simulink model "power_BLDC_EGR_Test"  (R2013b)
settings: Solver=FixedStepDiscrete  StartTime=0.0  StopTime=2  FixedStep=Ts  RelTol=1e-3
values from neighbouring files (symbols this model uses):
  C_BLDCM_POLE_NUM = 4    [EGR_Model_Init.m]
  C_BLDCM_ROTOR_RAD_INIT = Simulink.Parameter    [EGR_Model_Init.m]
  C_EGR_BLDC_STEP = 60    [EGR_Model_Init.m]
  C_EGR_BLDC_VALVE_SCREW_LOAD_PITCH = 4    [EGR_Model_Init.m]
  K_BLDCM_DAMPING_COEFF = Simulink.Parameter    [EGR_Model_Init.m]
  K_BLDCM_FLUX = Simulink.Parameter    [EGR_Model_Init.m]
  K_BLDCM_INDUCTANCE = Simulink.Parameter    [EGR_Model_Init.m]
  K_BLDCM_INERTIA = Simulink.Parameter    [EGR_Model_Init.m]
  K_BLDCM_RESISTANCE = Simulink.Parameter    [EGR_Model_Init.m]
  K_BLDCM_TF = Simulink.Parameter    [EGR_Model_Init.m]
  K_EGR_BLDC_LCD_POS_OFFSET = 0    [EGR_Model_Init.m]
  K_EGR_BLDC_VALVE_HS_RAD_HIGH = 15.9082    [EGR_Model_Init.m]
  K_EGR_BLDC_VALVE_HS_RAD_LOW = -3.27    [EGR_Model_Init.m]
  K_EGR_BLDC_VALVE_POS_RAD_INIT = 0    [EGR_Model_Init.m]
  K_EGR_BLDC_VALVE_POS_RAD_OFFSET = 1.047    [EGR_Model_Init.m]
  K_EGR_BLDC_VALVE_STOPPER_RAD = 0.2617    [EGR_Model_Init.m]
  K_EGR_SPRING_COEFF = Simulink.Parameter    [EGR_Model_Init.m]
  K_EGR_SPRING_TORQUE_COMP = 0    [EGR_Model_Init.m]
  Ts = 1e-4    (= 0.0001)    [EGR_Model_Init.m]
undefined symbols (not defined in the file or in its folder): DiscIntNeverNeededParam
settings Model: FPTRunName=FPA_Reference  TunableVars=EGR_BLDC_STEP,Ksp,egr_bldc_initpos,egr_pos_lower_limit,egr_pos_upper_limit,spring_compensation,spring_initpos,spring_maxpos  TunableVarsStorageClass=Auto,Auto,Auto,Auto,Auto,Auto,Auto,Auto  TunableVarsTypeQualifier=,,,,,,,  Creator=stoup_000  LastModifiedBy=TTI1783
settings DataIOCC: ExternalInput=[time2,input2]  SaveFormat=StructureWithTime  SignalLoggingSaveFormat=ModelDataLogs
settings OptimizationCC: InlineParams=on  UseFloatMulNetSlope=on  UseSpecifiedMinMax=on  InlineInvariantSignals=on  EnhancedBackFolding=on  ZeroExternalMemoryAtStartup=off  ZeroInternalMemoryAtStartup=off  EfficientFloat2IntCast=on  OptimizeModelRefInitCode=on  LifeSpan=1  MaxStackSize=64
settings DebuggingCC: MergeDetectMultiDrivingBlocksExec=error  ParameterPrecisionLossMsg=none
settings HardwareCC: ProdLargestAtomicInteger=Long  ProdLargestAtomicFloat=Double  ProdEndianess=LittleEndian  ProdHWDeviceType=ARM Compatible->ARM Cortex
settings RTWCC: SystemTargetFile=ert.tlc  GenCodeOnly=on  GenerateMakefile=off  TemplateMakefile=ert_default_tmf  Description=Embedded Coder  GenerateReport=on  ProcessScript=ert_make_rtw_hook  Toolchain=GNU Tools for ARM Embedded Processors  IncludeHyperlinkInReport=on  LaunchReport=on  GenerateTraceInfo=on  GenerateTraceReport=on  GenerateTraceReportSl=on  GenerateTraceReportSf=on  GenerateTraceReportEml=on  RTWCompilerOptimization=On
settings CodeAppCC: ForceParamTrailComments=on  IgnoreCustomStorageClasses=off  IgnoreTestpoints=on  OperatorAnnotations=on  SimulinkDataObjDesc=on  SFDataObjDesc=on  MATLABFcnDesc=on  InsertBlockDesc=on  MATLABSourceComments=on  EnableCustomComments=on  ReqsInCode=on
settings ERTTargetCC: CodeReplacementLibrary=ANSI_C  GenerateSampleERTMain=on  IncludeMdlTerminateFcn=off  CombineSignalStateStructs=on  SuppressErrorStatus=on  SupportNonFinite=off  ERTCustomFileTemplate=example_file_process.tlc  ConvertIfToSwitch=on  SuppressUnreachableDefaultCases=on

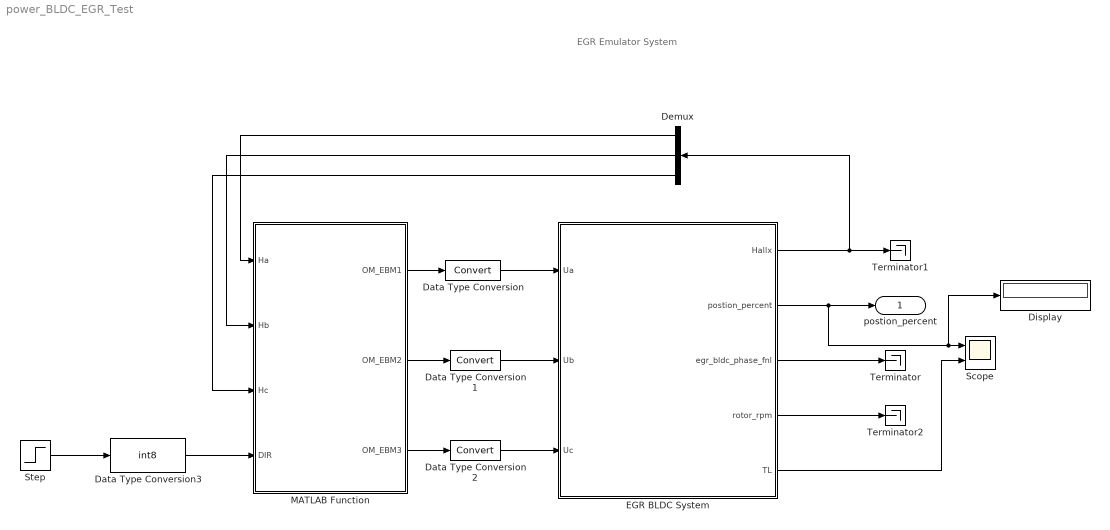
== system power_BLDC_EGR_Test ==
  note: EGR Emulator System
  Data Type Conversion : DataTypeConversion
  Data Type Conversion1 : DataTypeConversion
  Data Type Conversion2 : DataTypeConversion
  Data Type Conversion3 : DataTypeConversion  OutDataTypeStr=int8
  Demux : Demux  Outputs=3
  Display : Display
  EGR BLDC System : Subsystem  MinMaxOverflowLogging=MinMaxAndOverflow
  MATLAB Function : MATLAB Function  TreatAsAtomicUnit=on
  Scope : Scope  NumInputPorts=2
      settings: YMin=-5~-5  YMax=5~5
  Step : Step  Time=.5  Before=1  After=2  SampleTime=0
  Terminator : Terminator
  Terminator1 : Terminator
  Terminator2 : Terminator
  postion_percent : Outport
  wires:
  Data Type Conversion2/1 -> EGR BLDC System/3(Uc)
  Data Type Conversion1/1 -> EGR BLDC System/2(Ub)
  Data Type Conversion/1 -> EGR BLDC System/1(Ua)
  EGR BLDC System/2(postion_percent) -> Display/1, Scope/1, postion_percent/1
  Data Type Conversion3/1 -> MATLAB Function/4(DIR)
  MATLAB Function/1(OM_EBM1) -> Data Type Conversion/1
  MATLAB Function/2(OM_EBM2) -> Data Type Conversion1/1
  MATLAB Function/3(OM_EBM3) -> Data Type Conversion2/1
  EGR BLDC System/3(egr_bldc_phase_fnl) -> Terminator/1
  Demux/1 -> MATLAB Function/1(Ha)
  Demux/2 -> MATLAB Function/2(Hb)
  Demux/3 -> MATLAB Function/3(Hc)
  Step/1 -> Data Type Conversion3/1
  EGR BLDC System/1(Hallx) -> Demux/1, Terminator1/1
  EGR BLDC System/5(TL) -> Scope/2
  EGR BLDC System/4(rotor_rpm) -> Terminator2/1

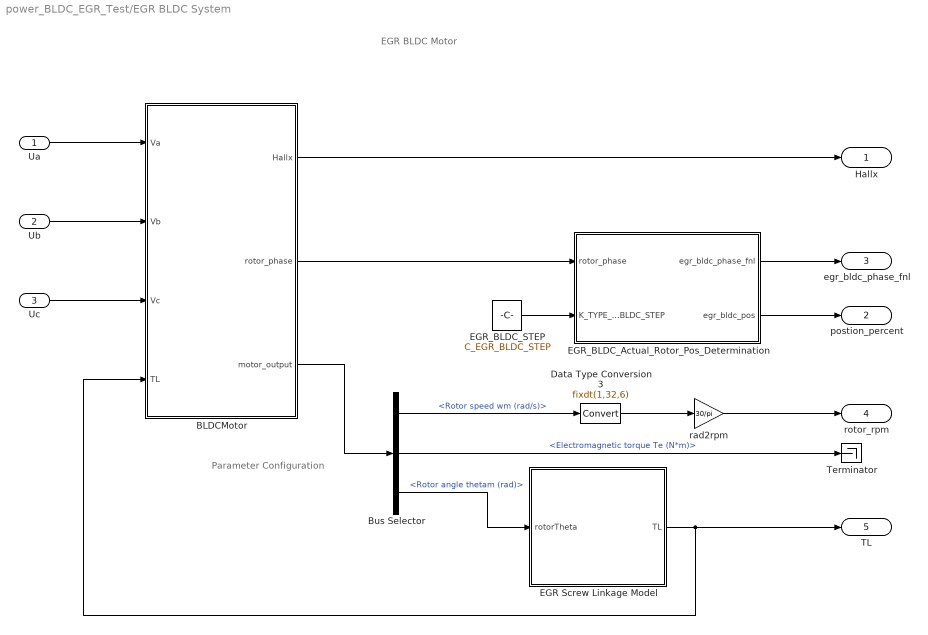
== system power_BLDC_EGR_Test/EGR BLDC System ==
  note: EGR BLDC Motor
  note: Parameter
      | Configuration
  Ua : Inport  OutDataTypeStr=fixdt(1,32,10)
  Ub : Inport  Port=2  OutDataTypeStr=fixdt(1,32,10)
  Uc : Inport  Port=3  OutDataTypeStr=fixdt(1,32,10)
  BLDCMotor : Subsystem
  Bus Selector : BusSelector  OutputSignals=Rotor speed wm (rad/s),Electromagnetic torque Te (N*m),Rotor angle thetam (rad)
  Data Type Conversion3 : DataTypeConversion  OutMin=-2000  OutMax=2000  OutDataTypeStr=fixdt(1,32,6)  RndMeth=Simplest
  EGR Screw Linkage Model : Subsystem  MinMaxOverflowLogging=MinMaxAndOverflow
  EGR_BLDC_Actual_Rotor_Pos_Determination : Subsystem  MinMaxOverflowLogging=MinMaxAndOverflow
  EGR_BLDC_STEP : Constant  Value=C_EGR_BLDC_STEP  OutDataTypeStr=uint8
  Terminator : Terminator
  rad2rpm : Gain  Gain=30/pi  ParamDataTypeStr=fixdt(1,32,10)  OutDataTypeStr=fixdt(1,32,10)  RndMeth=Simplest
  Hallx : Outport
  postion_percent : Outport  Port=2
  egr_bldc_phase_fnl : Outport  Port=3
  rotor_rpm : Outport  Port=4
  TL : Outport  Port=5
  wires:
  EGR Screw Linkage Model/1(TL) -> TL/1, BLDCMotor/4(TL)
  BLDCMotor/1(Hallx) -> Hallx/1
  rad2rpm/1 -> rotor_rpm/1
  Ua/1 -> BLDCMotor/1(Va)
  Ub/1 -> BLDCMotor/2(Vb)
  Uc/1 -> BLDCMotor/3(Vc)
  EGR_BLDC_STEP/1 -> EGR_BLDC_Actual_Rotor_Pos_Determination/2(K_TYPE_EGR_BLDC_STEP)
  EGR_BLDC_Actual_Rotor_Pos_Determination/2(egr_bldc_pos) -> postion_percent/1
  EGR_BLDC_Actual_Rotor_Pos_Determination/1(egr_bldc_phase_fnl) -> egr_bldc_phase_fnl/1
  Data Type Conversion3/1 -> rad2rpm/1
  BLDCMotor/2(rotor_phase) -> EGR_BLDC_Actual_Rotor_Pos_Determination/1(rotor_phase)
  BLDCMotor/3(motor_output) -> Bus Selector/1
  Bus Selector/1 -> Data Type Conversion3/1  "<Rotor speed wm (rad/s)>"
  Bus Selector/2 -> Terminator/1  "<Electromagnetic torque Te (N*m)>"
  Bus Selector/3 -> EGR Screw Linkage Model/1(rotorTheta)  "<Rotor angle thetam (rad)>"

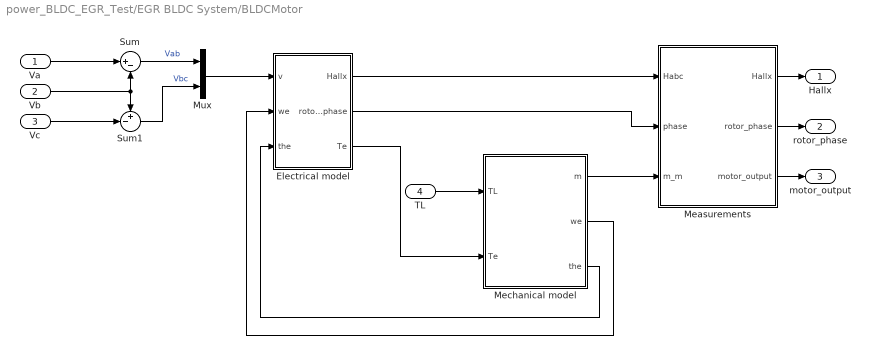
== system power_BLDC_EGR_Test/EGR BLDC System/BLDCMotor ==
  Va : Inport  OutDataTypeStr=fixdt(1,32,10)
  Vb : Inport  Port=2  OutDataTypeStr=fixdt(1,32,10)
  Vc : Inport  Port=3  OutDataTypeStr=fixdt(1,32,10)
  TL : Inport  Port=4  OutDataTypeStr=fixdt(1,32,10)
  Electrical model : Subsystem
  Measurements : Subsystem
  Mechanical model : Subsystem
  Mux : Mux  Inputs=2
  Sum : Sum  Inputs=|+-  OutDataTypeStr=fixdt(1,32,10)
  Sum1 : Sum  Inputs=+-|  OutDataTypeStr=fixdt(1,32,10)
  Hallx : Outport
  rotor_phase : Outport  Port=2
  motor_output : Outport  Port=3
  wires:
  Mechanical model/3(the) -> Electrical model/3(the)
  Mechanical model/1(m) -> Measurements/3(m_m)
  Mux/1 -> Electrical model/1(v)
  TL/1 -> Mechanical model/1(TL)
  Mechanical model/2(we) -> Electrical model/2(we)
  Electrical model/3(Te) -> Mechanical model/2(Te)
  Sum/1 -> Mux/1  "Vab"
  Va/1 -> Sum/1
  Vc/1 -> Sum1/2
  Sum1/1 -> Mux/2  "Vbc"
  Vb/1 -> Sum1/1, Sum/2
  Measurements/1(Hallx) -> Hallx/1
  Electrical model/1(Hallx) -> Measurements/1(Habc)
  Electrical model/2(rotor_phase) -> Measurements/2(phase)
  Measurements/2(rotor_phase) -> rotor_phase/1
  Measurements/3(motor_output) -> motor_output/1

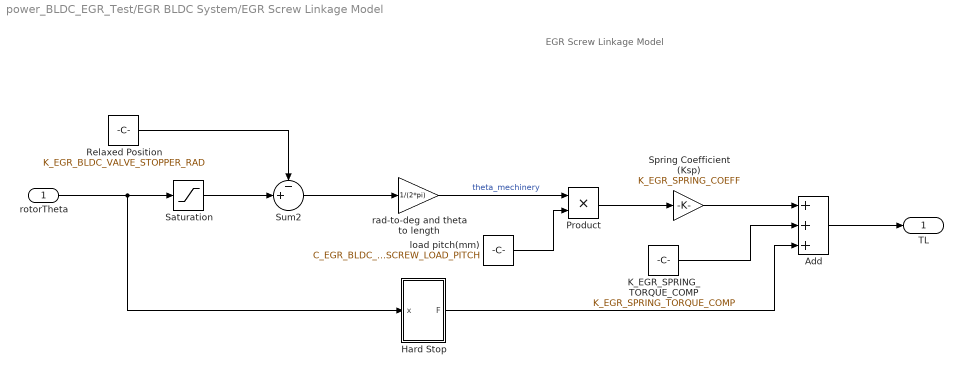
== system power_BLDC_EGR_Test/EGR BLDC System/EGR Screw Linkage Model ==
  note: EGR Screw Linkage Model
  rotorTheta : Inport  OutDataTypeStr=fixdt(1,32,10)
  Add : Sum  Inputs=+++  OutDataTypeStr=fixdt(1,32,10)
  Hard Stop : Subsystem
  K_EGR_SPRING_TORQUE_COMP : Constant  Value=K_EGR_SPRING_TORQUE_COMP  OutDataTypeStr=fixdt(1,32,10)
  Product : Product  OutDataTypeStr=fixdt(1,16,7)
  Relaxed Position : Constant  Value=K_EGR_BLDC_VALVE_STOPPER_RAD  OutDataTypeStr=fixdt(1,32,10)
  Saturation : Saturate  UpperLimit=K_EGR_BLDC_VALVE_HS_RAD_HIGH  LowerLimit=K_EGR_BLDC_VALVE_STOPPER_RAD  OutDataTypeStr=fixdt(1,32,10)
  Spring Coefficient (Ksp) : Gain  Gain=K_EGR_SPRING_COEFF  ParamDataTypeStr=fixdt(1,16,10)  OutDataTypeStr=fixdt(1,16,7)
  Sum2 : Sum  Inputs=-+|  OutDataTypeStr=fixdt(1,32,10)
  load pitch(mm) : Constant  Value=C_EGR_BLDC_VALVE_SCREW_LOAD_PITCH  OutDataTypeStr=fixdt(1,16,7)
  "rad-to-deg and theta to length " : Gain  Gain=1/(2*pi)  ParamDataTypeStr=fixdt(1,32,10)  OutDataTypeStr=fixdt(1,32,10)
  TL : Outport
  wires:
  Spring Coefficient (Ksp)/1 -> Add/1
  rotorTheta/1 -> Hard Stop/1(x), Saturation/1
  Relaxed Position/1 -> Sum2/1
  "rad-to-deg and theta to length "/1 -> Product/1  "theta_mechinery"
  load pitch(mm)/1 -> Product/2
  Sum2/1 -> "rad-to-deg and theta to length "/1
  Product/1 -> Spring Coefficient (Ksp)/1
  K_EGR_SPRING_TORQUE_COMP/1 -> Add/2
  Hard Stop/1(F) -> Add/3
  Add/1 -> TL/1
  Saturation/1 -> Sum2/2

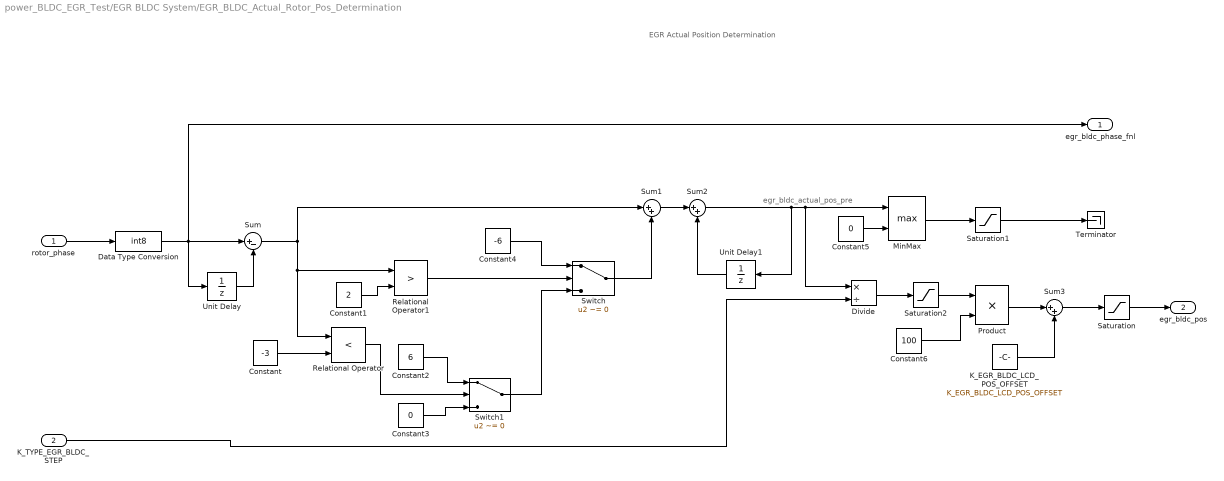
== system power_BLDC_EGR_Test/EGR BLDC System/EGR_BLDC_Actual_Rotor_Pos_Determination ==
  note: EGR Actual Position Determination
  note: egr_bldc_actual_pos_pre
  rotor_phase : Inport  OutDataTypeStr=int8
  K_TYPE_EGR_BLDC_STEP : Inport  Port=2  OutDataTypeStr=uint8
  Constant : Constant  Value=-3  OutDataTypeStr=int8
  Constant1 : Constant  Value=2  OutDataTypeStr=int8
  Constant2 : Constant  Value=6  OutDataTypeStr=int8
  Constant3 : Constant  Value=0  OutDataTypeStr=int8
  Constant4 : Constant  Value=-6  OutDataTypeStr=int8
  Constant5 : Constant  Value=0  OutDataTypeStr=uint8
  Constant6 : Constant  Value=100  OutDataTypeStr=uint8
  Data Type Conversion : DataTypeConversion  OutDataTypeStr=int8
  Divide : Product  Inputs=*/  OutDataTypeStr=fixdt(1,32,12)  RndMeth=Simplest
  K_EGR_BLDC_LCD_POS_OFFSET : Constant  Value=K_EGR_BLDC_LCD_POS_OFFSET  OutDataTypeStr=fixdt(1,16,7)
  MinMax : MinMax  Function=max  Inputs=2  OutDataTypeStr=fixdt(1,16,0)  SaturateOnIntegerOverflow=on
  Product : Product  OutDataTypeStr=fixdt(1,16,7)
  Relational Operator : RelationalOperator  Operator=<  OutDataTypeStr=boolean
  Relational Operator1 : RelationalOperator  Operator=>  OutDataTypeStr=boolean
  Saturation : Saturate  UpperLimit=125  LowerLimit=-25  OutDataTypeStr=fixdt(1,16,7)
  Saturation1 : Saturate  UpperLimit=120  LowerLimit=-60  OutDataTypeStr=int8
  Saturation2 : Saturate  UpperLimit=1.25  LowerLimit=-0.25  OutDataTypeStr=fixdt(1,16,12)
  Sum : Sum  Inputs=|+-  AccumDataTypeStr=int8  OutDataTypeStr=int8
  Sum1 : Sum  Inputs=|++  AccumDataTypeStr=int8  OutDataTypeStr=fixdt(1,8,0)
  Sum2 : Sum  Inputs=|++  AccumDataTypeStr=fixdt(1,16,0)  OutDataTypeStr=fixdt(1,16,0)
  Sum3 : Sum  Inputs=|++  OutDataTypeStr=fixdt(1,16,7)
  Switch : Switch  Criteria=u2 ~= 0  OutDataTypeStr=int8
  Switch1 : Switch  Criteria=u2 ~= 0  OutDataTypeStr=int8
  Terminator : Terminator
  Unit Delay : UnitDelay  SampleTime=-1
  Unit Delay1 : UnitDelay  SampleTime=-1
  egr_bldc_phase_fnl : Outport
  egr_bldc_pos : Outport  Port=2
  wires:
  MinMax/1 -> Saturation1/1
  Switch1/1 -> Switch/3
  Constant4/1 -> Switch/1
  Constant2/1 -> Switch1/1
  Constant/1 -> Relational Operator/2
  Constant3/1 -> Switch1/3
  Constant6/1 -> Product/2
  Relational Operator1/1 -> Switch/2
  Switch/1 -> Sum1/2
  Constant5/1 -> MinMax/2
  Relational Operator/1 -> Switch1/2
  Constant1/1 -> Relational Operator1/2
  Sum1/1 -> Sum2/1
  Unit Delay1/1 -> Sum2/2
  Sum/1 -> Relational Operator/1, Relational Operator1/1, Sum1/1
  Unit Delay/1 -> Sum/2
  Saturation1/1 -> Terminator/1
  K_EGR_BLDC_LCD_POS_OFFSET/1 -> Sum3/2
  Saturation/1 -> egr_bldc_pos/1
  Product/1 -> Sum3/1
  Sum3/1 -> Saturation/1
  Data Type Conversion/1 -> Unit Delay/1, egr_bldc_phase_fnl/1, Sum/1
  Sum2/1 -> Unit Delay1/1, Divide/1, MinMax/1
  rotor_phase/1 -> Data Type Conversion/1
  K_TYPE_EGR_BLDC_STEP/1 -> Divide/2
  Divide/1 -> Saturation2/1
  Saturation2/1 -> Product/1

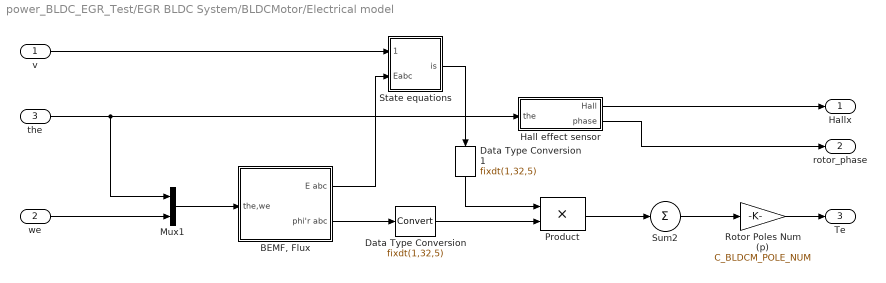
== system power_BLDC_EGR_Test/EGR BLDC System/BLDCMotor/Electrical model ==
  v : Inport
  we : Inport  Port=2
  the : Inport  Port=3
  "BEMF, Flux" : Subsystem
  Data Type Conversion : DataTypeConversion  OutDataTypeStr=fixdt(1,32,5)  RndMeth=Simplest
  Data Type Conversion1 : DataTypeConversion  OutDataTypeStr=fixdt(1,32,5)  RndMeth=Simplest
  Hall effect sensor : Subsystem
  Mux1 : Mux  Inputs=2
  Product : Product  OutDataTypeStr=fixdt(1,32,10)
  Rotor Poles Num (p) : Gain  Gain=C_BLDCM_POLE_NUM  ParamDataTypeStr=int8  OutDataTypeStr=fixdt(1,32,10)
  State equations : Subsystem
  Sum2 : Sum  Inputs=+  OutDataTypeStr=fixdt(1,32,10)  SaturateOnIntegerOverflow=on
  Hallx : Outport  OutDataTypeStr=boolean  InitialOutput=0
  rotor_phase : Outport  Port=2  InitialOutput=0
  Te : Outport  Port=3  OutDataTypeStr=fixdt(1,32,10)  InitialOutput=0
  wires:
  v/1 -> State equations/1(Vab,Vbc)
  Rotor Poles Num (p)/1 -> Te/1
  Sum2/1 -> Rotor Poles Num (p)/1
  "BEMF, Flux"/2(phi'r abc) -> Data Type Conversion/1
  Mux1/1 -> "BEMF, Flux"/1(the,we)
  Product/1 -> Sum2/1
  State equations/1(is) -> Data Type Conversion1/1
  "BEMF, Flux"/1(E abc) -> State equations/2(Eabc)
  we/1 -> Mux1/2
  Data Type Conversion/1 -> Product/2
  Data Type Conversion1/1 -> Product/1
  Hall effect sensor/1(Hall) -> Hallx/1
  Hall effect sensor/2(phase) -> rotor_phase/1
  the/1 -> Hall effect sensor/1(the), Mux1/1

== system power_BLDC_EGR_Test/EGR BLDC System/BLDCMotor/Measurements ==
  Habc : Inport  OutDataTypeStr=boolean
  phase : Inport  Port=2  OutDataTypeStr=int8
  m_m : Inport  Port=3  OutDataTypeStr=fixdt(1,32,10)
  Bus Creator1 : BusCreator  Inputs=3
  Demux1 : Demux  Outputs=[1,1,1]
  Hallx : Outport
  rotor_phase : Outport  Port=2
  motor_output : Outport  Port=3
  wires:
  Demux1/2 -> Bus Creator1/2  "Rotor angle thetam (rad)"
  Demux1/3 -> Bus Creator1/3  "Electromagnetic torque Te (N*m)"
  Demux1/1 -> Bus Creator1/1  "Rotor speed wm (rad/s)"
  m_m/1 -> Demux1/1
  Habc/1 -> Hallx/1
  phase/1 -> rotor_phase/1
  Bus Creator1/1 -> motor_output/1

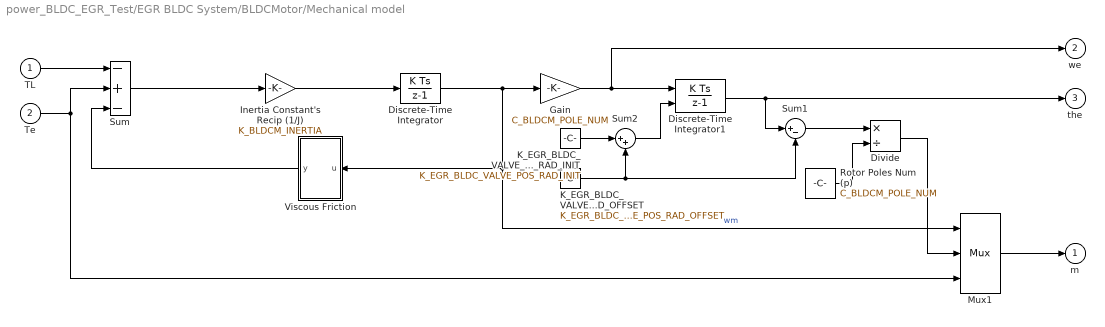
== system power_BLDC_EGR_Test/EGR BLDC System/BLDCMotor/Mechanical model ==
  TL : Inport
  Te : Inport  Port=2  OutDataTypeStr=fixdt(1,32,10)
  Discrete-Time Integrator : DiscreteIntegrator  InitialCondition=C_BLDCM_ROTOR_RAD_INIT  SampleTime=Ts  OutDataTypeStr=fixdt(1,32,10)  ICPrevOutput=DiscIntNeverNeededParam  ICPrevScaledInput=DiscIntNeverNeededParam
  Discrete-Time Integrator1 : DiscreteIntegrator  InitialConditionSource=external  SampleTime=Ts  OutDataTypeStr=fixdt(1,32,10)  ICPrevOutput=DiscIntNeverNeededParam  ICPrevScaledInput=DiscIntNeverNeededParam
  Divide : Product  Inputs=*/  OutDataTypeStr=fixdt(1,32,10)  RndMeth=Simplest
  Gain : Gain  Gain=C_BLDCM_POLE_NUM  ParamMin=0  ParamMax=10  ParamDataTypeStr=int8  OutDataTypeStr=fixdt(1,32,10)
  Inertia Constant's Recip (1/J) : Gain  Gain=K_BLDCM_INERTIA  ParamDataTypeStr=fixdt(1,32,10)  OutDataTypeStr=fixdt(1,32,10)
  K_EGR_BLDC_VALVE_POS_RAD_INIT : Constant  Value=K_EGR_BLDC_VALVE_POS_RAD_INIT  OutDataTypeStr=fixdt(1,32,10)
  K_EGR_BLDC_VALVE_POS_RAD_OFFSET : Constant  Value=K_EGR_BLDC_VALVE_POS_RAD_OFFSET  OutDataTypeStr=fixdt(1,32,10)
  Mux1 : Mux  Inputs=3
  Rotor Poles Num (p) : Constant  Value=C_BLDCM_POLE_NUM  OutDataTypeStr=int8
  Sum : Sum  Inputs=-+-  OutDataTypeStr=fixdt(1,32,10)  SaturateOnIntegerOverflow=on
  Sum1 : Sum  Inputs=|+-  OutDataTypeStr=fixdt(1,32,10)  RndMeth=Simplest
  Sum2 : Sum  Inputs=|++  OutDataTypeStr=fixdt(1,32,10)
  Viscous Friction : Subsystem
  m : Outport  OutDataTypeStr=fixdt(1,32,10)  InitialOutput=0
  we : Outport  Port=2  InitialOutput=0
  the : Outport  Port=3  InitialOutput=0
  wires:
  Te/1 -> Sum/2, Mux1/3
  Gain/1 -> we/1, Discrete-Time Integrator1/1
  Viscous Friction/1(y) -> Sum/3
  TL/1 -> Sum/1
  Discrete-Time Integrator/1 -> Mux1/1, Viscous Friction/1(u), Gain/1  "wm"
  Mux1/1 -> m/1
  Divide/1 -> Mux1/2
  K_EGR_BLDC_VALVE_POS_RAD_OFFSET/1 -> Sum2/2, Sum1/2
  Sum1/1 -> Divide/1
  Sum/1 -> Inertia Constant's Recip (1/J)/1
  Inertia Constant's Recip (1/J)/1 -> Discrete-Time Integrator/1
  Discrete-Time Integrator1/1 -> Sum1/1, the/1
  K_EGR_BLDC_VALVE_POS_RAD_INIT/1 -> Sum2/1
  Sum2/1 -> Discrete-Time Integrator1/2
  Rotor Poles Num (p)/1 -> Divide/2

== system power_BLDC_EGR_Test/EGR BLDC System/EGR Screw Linkage Model/Hard Stop ==
  note: Spring Hard Stop
  x : Inport
  Gain2 : Gain  Gain=800  OutDataTypeStr=fixdt(1,32,10)  ParamDataTypeStr=Inherit: Same as input
  High : Constant  Value=K_EGR_BLDC_VALVE_HS_RAD_HIGH  OutDataTypeStr=fixdt(1,32,10)
  Low : Constant  Value=K_EGR_BLDC_VALVE_HS_RAD_LOW  OutDataTypeStr=fixdt(1,32,10)
  Min1 : MinMax  Inputs=2  OutDataTypeStr=fixdt(1,32,10)  SaturateOnIntegerOverflow=on
  Min3 : MinMax  Function=max  Inputs=2  OutDataTypeStr=fixdt(1,32,10)  SaturateOnIntegerOverflow=on
  Sum5 : Sum  Inputs=-+||+-  OutDataTypeStr=fixdt(1,32,10)  SaturateOnIntegerOverflow=on
  F : Outport
  wires:
  Sum5/1 -> Gain2/1
  x/1 -> Min3/2, Min1/1
  Gain2/1 -> F/1
  Min3/1 -> Sum5/2
  Low/1 -> Sum5/4, Min1/2
  High/1 -> Min3/1, Sum5/1
  Min1/1 -> Sum5/3

== system power_BLDC_EGR_Test/EGR BLDC System/BLDCMotor/Electrical model/BEMF, Flux ==
  the,we : Inport
  Mux4 : Mux  Inputs=3
  Mux7 : Mux  Inputs=3
  Phase a : Subsystem
  Phase b : Subsystem
  Phase c : Subsystem
  E abc : Outport  OutDataTypeStr=fixdt(1,32,10)
  phi'r abc : Outport  Port=2  OutDataTypeStr=fixdt(1,32,10)
  wires:
  Mux7/1 -> phi'r abc/1
  Mux4/1 -> E abc/1
  Phase c/1(phi'r) -> Mux7/3
  Phase b/1(phi'r) -> Mux7/2
  Phase a/1(phi'r) -> Mux7/1
  Phase c/2(E) -> Mux4/3
  Phase b/2(E) -> Mux4/2
  Phase a/2(E) -> Mux4/1
  the,we/1 -> Phase b/1(the,we), Phase a/1(the,we), Phase c/1(the,we)

== system power_BLDC_EGR_Test/EGR BLDC System/BLDCMotor/Electrical model/Hall effect sensor ==
  note: BLDC Motor Hall Encoder
  the : Inport
  S-Function HallDecoder : S-Function  InitFcn=try, set_param(gcb,'FunctionName','HallEncoder'), end  FunctionName=HallEncoder  SFunctionModules=HallEncoder_wrapper  EnableBusSupport=off  mask(S-Function Builder){}
      mask help: Simulink:masks:SFunctionBuilder_MD
      mask init:
      | val = [[.9  0.75 0.75 1 1 .9 .9 1]',[1 1 0.75 0.75 .9 .9 1 .9]'];try , sys = get_param(gcb,'SfunBuilderFcnName');if isempty(sys), sys = get_param(gcb,'FunctionName'); end,catch, sys = get_param(gcb,'FunctionName'); end
      settings: CopyFcn=set_param(gcbh,'LinkStatus','none')  PreSaveFcn=try, set_param(gcb,'FunctionName','HallEncoder'), end  OpenFcn=sfunctionwizard(gcbh)
      mask Display: plot(val(:,1),val(:,2)),disp(sys), port_label('input',1,'theta'), port_label('output',1,'Hallx'), port_label('output',2,'phase')
  rad2deg1 : Gain  Gain=180/pi  OutMin=-360  OutMax=360  OutDataTypeStr=double  RndMeth=Simplest
  rem : Subsystem  TreatAsAtomicUnit=on
  Hall : Outport  OutDataTypeStr=boolean
  phase : Outport  Port=2  OutDataTypeStr=int8
  wires:
  S-Function HallDecoder/1 -> Hall/1
  S-Function HallDecoder/2 -> phase/1
  the/1 -> rem/1(the)
  rem/1(rad) -> rad2deg1/1
  rad2deg1/1 -> S-Function HallDecoder/1

== system power_BLDC_EGR_Test/EGR BLDC System/BLDCMotor/Electrical model/State equations ==
  Vab,Vbc : Inport
  Eabc : Inport  Port=2  OutDataTypeStr=fixdt(1,32,10)
  Mux5 : Mux  Inputs=3
  State Ia : Subsystem
  State Ib : Subsystem
  Sum1 : Sum  Inputs=--  OutDataTypeStr=fixdt(1,32,10)  SaturateOnIntegerOverflow=on
  is : Outport  OutDataTypeStr=fixdt(1,32,10)
  wires:
  Mux5/1 -> is/1
  Eabc/1 -> State Ib/2(Eabc), State Ia/2(Eabc)
  Sum1/1 -> Mux5/3
  State Ia/1(i) -> Sum1/1, Mux5/1
  Vab,Vbc/1 -> State Ib/1(Vab,Vbc), State Ia/1(Vab,Vbc)
  State Ib/1(i) -> Sum1/2, Mux5/2

== system power_BLDC_EGR_Test/EGR BLDC System/BLDCMotor/Mechanical model/Viscous Friction ==
  note: y = sign(x) * (Gain * abs(x) + Offset)
  u : Inport
  Damping Constant (B) : Gain  Gain=K_BLDCM_DAMPING_COEFF  ParamDataTypeStr=fixdt(1,32,10)  OutDataTypeStr=fixdt(1,32,10)
  Shaft static friction torque (Tf) : Gain  Gain=K_BLDCM_TF  ParamDataTypeStr=fixdt(1,32,10)  OutDataTypeStr=fixdt(1,32,10)
  Sign : Signum  DisableCoverage=on
  Sum2 : Sum  Inputs=|++  SaturateOnIntegerOverflow=on  InputSameDT=on  OutDataTypeStr=Inherit: Same as first input
  y : Outport
  wires:
  Damping Constant (B)/1 -> Sum2/2
  Shaft static friction torque (Tf)/1 -> Sum2/1
  Sign/1 -> Shaft static friction torque (Tf)/1
  u/1 -> Damping Constant (B)/1, Sign/1
  Sum2/1 -> y/1

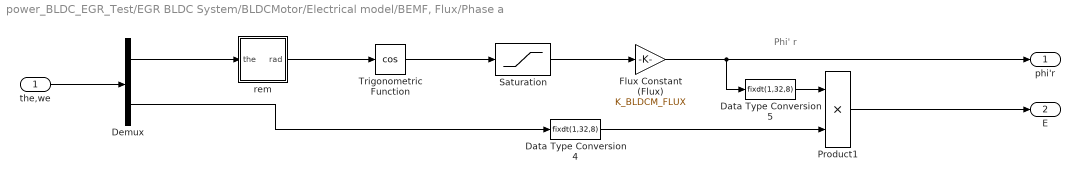
== system power_BLDC_EGR_Test/EGR BLDC System/BLDCMotor/Electrical model/BEMF, Flux/Phase a ==
  note: Phi' r
  the,we : Inport
  Data Type Conversion4 : DataTypeConversion  OutMin=-1000  OutMax=1000  OutDataTypeStr=fixdt(1,32,8)
  Data Type Conversion5 : DataTypeConversion  OutMin=-10  OutMax=10  OutDataTypeStr=fixdt(1,32,8)
  Demux : Demux  Outputs=2
  Flux Constant (Flux) : Gain  Gain=K_BLDCM_FLUX  ParamDataTypeStr=fixdt(1,32,10)  OutDataTypeStr=fixdt(1,32,10)
  Product1 : Product  OutDataTypeStr=fixdt(1,32,10)
  Saturation : Saturate  OutMin=-1  OutMax=1  OutDataTypeStr=fixdt(1,32,10)
  Trigonometric Function : Trigonometry  Operator=cos  ApproximationMethod=CORDIC
  rem : Subsystem  TreatAsAtomicUnit=on
  phi'r : Outport  OutDataTypeStr=fixdt(1,32,10)
  E : Outport  Port=2  OutDataTypeStr=fixdt(1,32,10)
  wires:
  Flux Constant (Flux)/1 -> phi'r/1, Data Type Conversion5/1
  the,we/1 -> Demux/1
  Demux/2 -> Data Type Conversion4/1
  Saturation/1 -> Flux Constant (Flux)/1
  Product1/1 -> E/1
  Data Type Conversion4/1 -> Product1/2
  Data Type Conversion5/1 -> Product1/1
  Demux/1 -> rem/1(the)
  Trigonometric Function/1 -> Saturation/1
  rem/1(rad) -> Trigonometric Function/1

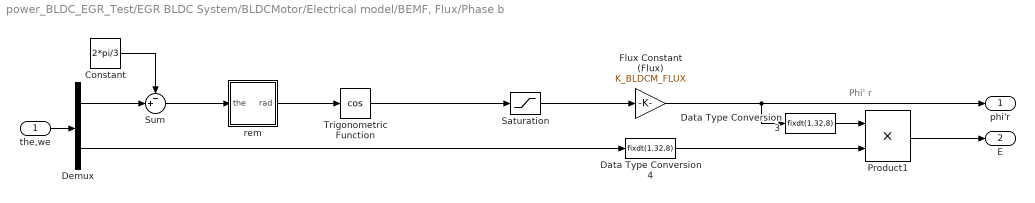
== system power_BLDC_EGR_Test/EGR BLDC System/BLDCMotor/Electrical model/BEMF, Flux/Phase b ==
  note: Phi' r
  the,we : Inport
  Constant : Constant  Value=2*pi/3  OutDataTypeStr=fixdt(1,32,29)
  Data Type Conversion3 : DataTypeConversion  OutMin=-10  OutMax=10  OutDataTypeStr=fixdt(1,32,8)
  Data Type Conversion4 : DataTypeConversion  OutMin=-1000  OutMax=1000  OutDataTypeStr=fixdt(1,32,8)
  Demux : Demux  Outputs=2
  Flux Constant (Flux) : Gain  Gain=K_BLDCM_FLUX  ParamDataTypeStr=fixdt(1,32,10)  OutDataTypeStr=fixdt(1,32,10)
  Product1 : Product  OutDataTypeStr=fixdt(1,32,10)
  Saturation : Saturate  OutMin=-1  OutMax=1  OutDataTypeStr=fixdt(1,32,10)
  Sum : Sum  Inputs=-+|  OutDataTypeStr=fixdt(1,32,10)
  Trigonometric Function : Trigonometry  Operator=cos  ApproximationMethod=CORDIC
  rem : Subsystem  TreatAsAtomicUnit=on
  phi'r : Outport  OutDataTypeStr=fixdt(1,32,10)
  E : Outport  Port=2  OutDataTypeStr=fixdt(1,32,10)
  wires:
  Saturation/1 -> Flux Constant (Flux)/1
  Demux/2 -> Data Type Conversion4/1
  the,we/1 -> Demux/1
  Product1/1 -> E/1
  Flux Constant (Flux)/1 -> phi'r/1, Data Type Conversion3/1
  Constant/1 -> Sum/1
  Demux/1 -> Sum/2
  Data Type Conversion4/1 -> Product1/2
  Data Type Conversion3/1 -> Product1/1
  Trigonometric Function/1 -> Saturation/1
  Sum/1 -> rem/1(the)
  rem/1(rad) -> Trigonometric Function/1

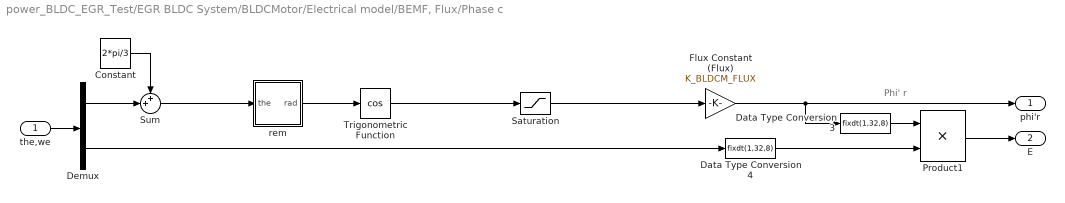
== system power_BLDC_EGR_Test/EGR BLDC System/BLDCMotor/Electrical model/BEMF, Flux/Phase c ==
  note: Phi' r
  the,we : Inport
  Constant : Constant  Value=2*pi/3  OutDataTypeStr=fixdt(1,32,29)
  Data Type Conversion3 : DataTypeConversion  OutMin=-10  OutMax=10  OutDataTypeStr=fixdt(1,32,8)
  Data Type Conversion4 : DataTypeConversion  OutMin=-1000  OutMax=1000  OutDataTypeStr=fixdt(1,32,8)
  Demux : Demux  Outputs=2
  Flux Constant (Flux) : Gain  Gain=K_BLDCM_FLUX  ParamDataTypeStr=fixdt(1,32,10)  OutDataTypeStr=fixdt(1,32,10)
  Product1 : Product  OutDataTypeStr=fixdt(1,32,10)
  Saturation : Saturate  OutMin=-1  OutMax=1  OutDataTypeStr=fixdt(1,32,10)
  Sum : Sum  Inputs=++|  OutDataTypeStr=fixdt(1,32,10)
  Trigonometric Function : Trigonometry  Operator=cos  ApproximationMethod=CORDIC
  rem : Subsystem  TreatAsAtomicUnit=on
  phi'r : Outport  OutDataTypeStr=fixdt(1,32,10)
  E : Outport  Port=2  OutDataTypeStr=fixdt(1,32,10)
  wires:
  Flux Constant (Flux)/1 -> phi'r/1, Data Type Conversion3/1
  Product1/1 -> E/1
  the,we/1 -> Demux/1
  Demux/2 -> Data Type Conversion4/1
  Demux/1 -> Sum/2
  Saturation/1 -> Flux Constant (Flux)/1
  Constant/1 -> Sum/1
  Data Type Conversion4/1 -> Product1/2
  Data Type Conversion3/1 -> Product1/1
  Sum/1 -> rem/1(the)
  Trigonometric Function/1 -> Saturation/1
  rem/1(rad) -> Trigonometric Function/1

== system power_BLDC_EGR_Test/EGR BLDC System/BLDCMotor/Electrical model/Hall effect sensor/rem ==
  the : Inport
  Constant : Constant  Value=2*pi  OutDataTypeStr=double
  Data Type Conversion : DataTypeConversion  OutDataTypeStr=double
  Data Type Conversion1 : DataTypeConversion  OutMin=-2*pi  OutMax=2*pi  OutDataTypeStr=fixdt(1,32,10)  RndMeth=Simplest
  S-Function Builder : S-Function  InitFcn=try, set_param(gcb,'FunctionName','remf'), end  FunctionName=remf  SFunctionModules=remf_wrapper  EnableBusSupport=off  mask(S-Function Builder){}
      mask help: Simulink:masks:SFunctionBuilder_MD
      mask init: same as power_BLDC_EGR_Test/EGR BLDC System/BLDCMotor/Electrical model/Hall effect sensor/S-Function HallDecoder
      settings: CopyFcn=set_param(gcbh,'LinkStatus','none')  PreSaveFcn=try, set_param(gcb,'FunctionName','remf'), end  OpenFcn=sfunctionwizard(gcbh)
      mask Display: plot(val(:,1),val(:,2)),disp(sys), port_label('input',1,'x'), port_label('input',2,'y'), port_label('output',1,'z')
  rad : Outport
  wires:
  Constant/1 -> S-Function Builder/2
  S-Function Builder/1 -> Data Type Conversion1/1
  the/1 -> Data Type Conversion/1
  Data Type Conversion/1 -> S-Function Builder/1
  Data Type Conversion1/1 -> rad/1

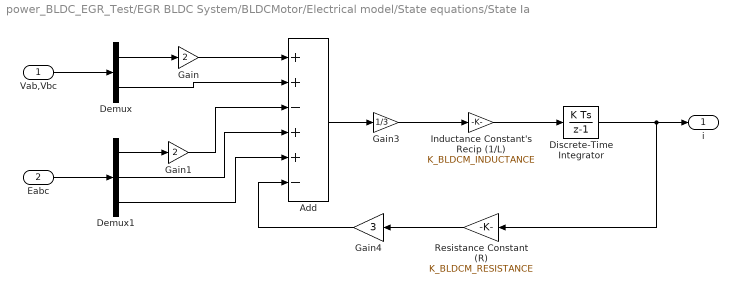
== system power_BLDC_EGR_Test/EGR BLDC System/BLDCMotor/Electrical model/State equations/State Ia ==
  Vab,Vbc : Inport  OutDataTypeStr=fixdt(1,32,10)
  Eabc : Inport  Port=2  OutDataTypeStr=fixdt(1,32,10)
  Add : Sum  Inputs=++-++-  OutDataTypeStr=fixdt(1,32,10)
  Demux : Demux  Outputs=2
  Demux1 : Demux  Outputs=3
  Discrete-Time Integrator : DiscreteIntegrator  SampleTime=Ts  OutDataTypeStr=fixdt(1,32,10)  ICPrevOutput=DiscIntNeverNeededParam  ICPrevScaledInput=DiscIntNeverNeededParam
  Gain : Gain  Gain=2  OutDataTypeStr=fixdt(1,32,10)
  Gain1 : Gain  Gain=2  OutDataTypeStr=fixdt(1,32,10)
  Gain3 : Gain  Gain=1/3  ParamDataTypeStr=fixdt(1,32,10)  OutDataTypeStr=fixdt(1,32,10)
  Gain4 : Gain  Gain=3  OutDataTypeStr=fixdt(1,32,10)  ParamDataTypeStr=Inherit: Same as input
  Inductance Constant's Recip (1/L) : Gain  Gain=K_BLDCM_INDUCTANCE  ParamDataTypeStr=fixdt(1,32,10)  OutDataTypeStr=fixdt(1,32,10)
  Resistance Constant (R) : Gain  Gain=K_BLDCM_RESISTANCE  ParamDataTypeStr=fixdt(1,32,10)  OutDataTypeStr=fixdt(1,32,10)
  i : Outport  OutDataTypeStr=fixdt(1,32,10)
  wires:
  Inductance Constant's Recip (1/L)/1 -> Discrete-Time Integrator/1
  Vab,Vbc/1 -> Demux/1
  Eabc/1 -> Demux1/1
  Demux/1 -> Gain/1
  Gain/1 -> Add/1
  Demux/2 -> Add/2
  Demux1/1 -> Gain1/1
  Gain1/1 -> Add/3
  Demux1/2 -> Add/4
  Demux1/3 -> Add/5
  Resistance Constant (R)/1 -> Gain4/1
  Discrete-Time Integrator/1 -> Resistance Constant (R)/1, i/1
  Add/1 -> Gain3/1
  Gain4/1 -> Add/6
  Gain3/1 -> Inductance Constant's Recip (1/L)/1

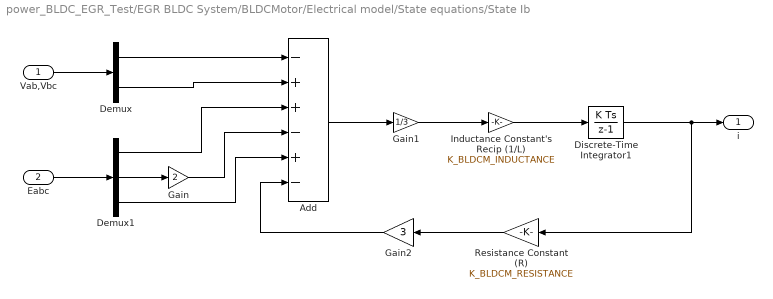
== system power_BLDC_EGR_Test/EGR BLDC System/BLDCMotor/Electrical model/State equations/State Ib ==
  Vab,Vbc : Inport
  Eabc : Inport  Port=2  OutDataTypeStr=fixdt(1,32,10)
  Add : Sum  Inputs=-++-+-  OutDataTypeStr=fixdt(1,32,10)
  Demux : Demux  Outputs=2
  Demux1 : Demux  Outputs=3
  Discrete-Time Integrator1 : DiscreteIntegrator  SampleTime=Ts  OutDataTypeStr=fixdt(1,32,10)  ICPrevOutput=DiscIntNeverNeededParam  ICPrevScaledInput=DiscIntNeverNeededParam
  Gain : Gain  Gain=2  OutDataTypeStr=fixdt(1,32,10)
  Gain1 : Gain  Gain=1/3  ParamDataTypeStr=fixdt(1,32,10)  OutDataTypeStr=fixdt(1,32,10)
  Gain2 : Gain  Gain=3  ParamDataTypeStr=int8  OutDataTypeStr=fixdt(1,32,10)
  Inductance Constant's Recip (1/L) : Gain  Gain=K_BLDCM_INDUCTANCE  ParamDataTypeStr=fixdt(1,32,10)  OutDataTypeStr=fixdt(1,32,10)
  Resistance Constant (R) : Gain  Gain=K_BLDCM_RESISTANCE  ParamDataTypeStr=fixdt(1,32,10)  OutDataTypeStr=fixdt(1,32,10)
  i : Outport  OutDataTypeStr=fixdt(1,32,10)
  wires:
  Vab,Vbc/1 -> Demux/1
  Eabc/1 -> Demux1/1
  Demux/2 -> Add/2
  Demux1/2 -> Gain/1
  Demux1/3 -> Add/5
  Gain2/1 -> Add/6
  Demux/1 -> Add/1
  Demux1/1 -> Add/3
  Gain/1 -> Add/4
  Inductance Constant's Recip (1/L)/1 -> Discrete-Time Integrator1/1
  Add/1 -> Gain1/1
  Discrete-Time Integrator1/1 -> Resistance Constant (R)/1, i/1
  Resistance Constant (R)/1 -> Gain2/1
  Gain1/1 -> Inductance Constant's Recip (1/L)/1

== system power_BLDC_EGR_Test/EGR BLDC System/BLDCMotor/Electrical model/BEMF, Flux/Phase a/rem ==
  the : Inport
  Constant : Constant  Value=2*pi  OutDataTypeStr=double
  Data Type Conversion : DataTypeConversion  OutDataTypeStr=double
  Data Type Conversion1 : DataTypeConversion  OutMin=-2*pi  OutMax=2*pi  OutDataTypeStr=fixdt(1,32,10)  RndMeth=Simplest
  S-Function Builder : S-Function  InitFcn=try, set_param(gcb,'FunctionName','remf'), end  FunctionName=remf  SFunctionModules=remf_wrapper  EnableBusSupport=off  mask(S-Function Builder){}
      mask help: Simulink:masks:SFunctionBuilder_MD
      mask init: same as power_BLDC_EGR_Test/EGR BLDC System/BLDCMotor/Electrical model/Hall effect sensor/S-Function HallDecoder
      settings: CopyFcn=set_param(gcbh,'LinkStatus','none')  PreSaveFcn=try, set_param(gcb,'FunctionName','remf'), end  OpenFcn=sfunctionwizard(gcbh)
      mask Display: plot(val(:,1),val(:,2)),disp(sys), port_label('input',1,'x'), port_label('input',2,'y'), port_label('output',1,'z')
  rad : Outport
  wires:
  Constant/1 -> S-Function Builder/2
  S-Function Builder/1 -> Data Type Conversion1/1
  the/1 -> Data Type Conversion/1
  Data Type Conversion/1 -> S-Function Builder/1
  Data Type Conversion1/1 -> rad/1

== system power_BLDC_EGR_Test/EGR BLDC System/BLDCMotor/Electrical model/BEMF, Flux/Phase b/rem ==
  the : Inport
  Constant : Constant  Value=2*pi  OutDataTypeStr=double
  Data Type Conversion : DataTypeConversion  OutDataTypeStr=double
  Data Type Conversion1 : DataTypeConversion  OutMin=-2*pi  OutMax=2*pi  OutDataTypeStr=fixdt(1,32,10)  RndMeth=Simplest
  S-Function Builder : S-Function  InitFcn=try, set_param(gcb,'FunctionName','remf'), end  FunctionName=remf  SFunctionModules=remf_wrapper  EnableBusSupport=off  mask(S-Function Builder){}
      mask help: Simulink:masks:SFunctionBuilder_MD
      mask init: same as power_BLDC_EGR_Test/EGR BLDC System/BLDCMotor/Electrical model/Hall effect sensor/S-Function HallDecoder
      settings: CopyFcn=set_param(gcbh,'LinkStatus','none')  PreSaveFcn=try, set_param(gcb,'FunctionName','remf'), end  OpenFcn=sfunctionwizard(gcbh)
      mask Display: plot(val(:,1),val(:,2)),disp(sys), port_label('input',1,'x'), port_label('input',2,'y'), port_label('output',1,'z')
  rad : Outport
  wires:
  Constant/1 -> S-Function Builder/2
  S-Function Builder/1 -> Data Type Conversion1/1
  the/1 -> Data Type Conversion/1
  Data Type Conversion/1 -> S-Function Builder/1
  Data Type Conversion1/1 -> rad/1

== system power_BLDC_EGR_Test/EGR BLDC System/BLDCMotor/Electrical model/BEMF, Flux/Phase c/rem ==
  the : Inport
  Constant : Constant  Value=2*pi  OutDataTypeStr=double
  Data Type Conversion : DataTypeConversion  OutDataTypeStr=double
  Data Type Conversion1 : DataTypeConversion  OutMin=-2*pi  OutMax=2*pi  OutDataTypeStr=fixdt(1,32,10)  RndMeth=Simplest
  S-Function Builder : S-Function  InitFcn=try, set_param(gcb,'FunctionName','remf'), end  FunctionName=remf  SFunctionModules=remf_wrapper  EnableBusSupport=off  mask(S-Function Builder){}
      mask help: Simulink:masks:SFunctionBuilder_MD
      mask init: same as power_BLDC_EGR_Test/EGR BLDC System/BLDCMotor/Electrical model/Hall effect sensor/S-Function HallDecoder
      settings: CopyFcn=set_param(gcbh,'LinkStatus','none')  PreSaveFcn=try, set_param(gcb,'FunctionName','remf'), end  OpenFcn=sfunctionwizard(gcbh)
      mask Display: plot(val(:,1),val(:,2)),disp(sys), port_label('input',1,'x'), port_label('input',2,'y'), port_label('output',1,'z')
  rad : Outport
  wires:
  Constant/1 -> S-Function Builder/2
  S-Function Builder/1 -> Data Type Conversion1/1
  the/1 -> Data Type Conversion/1
  Data Type Conversion/1 -> S-Function Builder/1
  Data Type Conversion1/1 -> rad/1

== matlab function power_BLDC_EGR_Test/MATLAB Function ==
  data: Ha input; OM_EBM1 output; Hb input; Hc input; OM_EBM2 output; OM_EBM3 output; DIR input
function [OM_EBM1, OM_EBM2, OM_EBM3] = ...
          fcn(Ha,Hb,Hc,DIR)
%#codegen
Voltage = 48;
switch(DIR)
    case 1 % Close Mode.
        if(Ha==1 && Hb==0 && Hc==1)
            OM_EBM1 = Voltage; 
            OM_EBM2 = 0;
            OM_EBM3 = Voltage/2;
        elseif(Ha==1 && Hb==0 && Hc==0)
            OM_EBM1 = Voltage; 
            OM_EBM2 = Voltage/2;
            OM_EBM3 = 0;
        elseif(Ha==1 && Hb==1 && Hc==0)
            OM_EBM1 = Voltage/2; 
            OM_EBM2 = Voltage;
            OM_EBM3 = 0;
        elseif(Ha==0 && Hb==1 && Hc==0)
            OM_EBM1 = 0; 
            OM_EBM2 = Voltage;
            OM_EBM3 = Voltage/2;
        elseif(Ha==0 && Hb==1 && Hc==1)
            OM_EBM1 = 0; 
            OM_EBM2 = Voltage/2;
            OM_EBM3 = Voltage;
        elseif(Ha==0 && Hb==0 && Hc==1)
            OM_EBM1 = Voltage/2; 
            OM_EBM2 = 0;
            OM_EBM3 = Voltage;
        else
            OM_EBM1 = 0; 
            OM_EBM2 = 0;
            OM_EBM3 = 0;
        end
      case 2 % Open Mode.
        if(Ha==1 && Hb==0 && Hc==1)
            OM_EBM1 = 0; 
            OM_EBM2 = Voltage;
            OM_EBM3 = Voltage/2;
        elseif(Ha==1 && Hb==0 && Hc==0)
            OM_EBM1 = 0; 
            OM_EBM2 = Voltage/2;
            OM_EBM3 = Voltage;
        elseif(Ha==1 && Hb==1 && Hc==0)
            OM_EBM1 = Voltage/2; 
            OM_EBM2 = 0;
            OM_EBM3 = Voltage;
        elseif(Ha==0 && Hb==1 && Hc==0)
            OM_EBM1 = Voltage; 
            OM_EBM2 = 0;
            OM_EBM3 = Voltage/2;
        elseif(Ha==0 && Hb==1 && Hc==1)
            OM_EBM1 = Voltage; 
            OM_EBM2 = Voltage/2;
            OM_EBM3 = 0;
        elseif(Ha==0 && Hb==0 && Hc==1)
            OM_EBM1 = Voltage/2; 
            OM_EBM2 = Voltage;
            OM_EBM3 = 0;
        else
            OM_EBM1 = 0; 
            OM_EBM2 = 0;
            OM_EBM3 = 0;
        end
    case 4 % brake mode
            OM_EBM1 = 0; 
            OM_EBM2 = 0;
            OM_EBM3 = 0;
    case 0 % Disable Mode
            OM_EBM1 = Voltage/2; 
            OM_EBM2 = Voltage/2;
            OM_EBM3 = Voltage/2;
    otherwise %Disable Mode
            OM_EBM1 = 0; 
            OM_EBM2 = 0;
            OM_EBM3 = 0;
end
